simulink model "PSK8_DigitalBandpassComm"  (R2019b)
settings: Solver=VariableStepAuto  StartTime=0.0  StopTime=1e-2  RelTol=1e-3
libraries: commutil2 x2, dspsrcs4 x2, commdigbbndpm3 x2, commfilt2 x2, commchan3 x1, commsink2 x1, commrandsrc3 x1
settings Model: Creator=SEFA  LastModifiedBy=SEFA

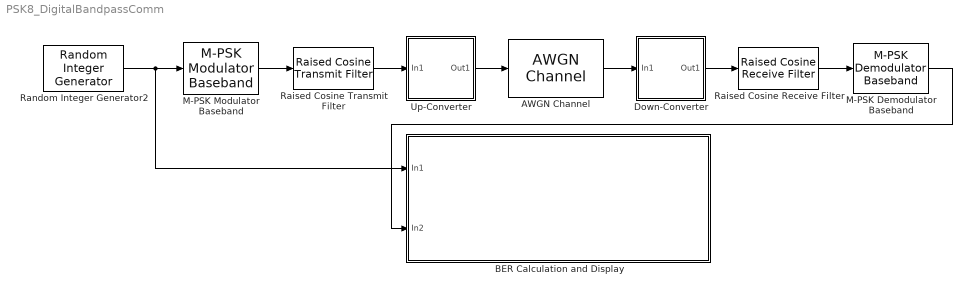
== system PSK8_DigitalBandpassComm ==
  AWGN Channel : commchan3/AWGN Channel  InputProcessing=Columns as channels (frame based)  seed=67  noiseMode="Signal to noise ratio  (Es/No)"  EbNodB=10  EsNodB=SNR  SNRdB=10  bitsPerSym=1  Ps=1/(16)  Tsym=1e-6  variance=1
      settings: SourceProductName=Communications Toolbox
  BER Calculation and Display : Subsystem
  Down-Converter : Subsystem
  M-PSK Demodulator Baseband : commdigbbndpm3/M-PSK Demodulator Baseband  M=8  OutType=Integer  DecType=Hard decision  VarSource=Dialog  Variance=1  Dec=Gray  Mapping=[0:7]  Ph=0  outDtype1=Inherit via internal rule  outDtype2=Inherit via internal rule  derotateFactorWordLen=16  derotateFactorDataTypeStr=Inherit: Same word length as input  derotateFactorLastDataTypeStr=Inherit: Same word length as input
      settings: SourceProductName=Communications Toolbox
  M-PSK Modulator Baseband : commdigbbndpm3/M-PSK Modulator Baseband  M=8  InType=Integer  Enc=Gray  Mapping=[0:7]  Ph=0  outDtype=double  outWordLen=16  outUDDataType=sfix(16)  outFracLenMode=Best precision  outFracLen=15  outDataTypeStr=double  outLastDataTypeStr=double
      settings: SourceProductName=Communications Toolbox
  Raised Cosine Receive Filter : commfilt2/Raised Cosine Receive Filter  filtType=Square root  R=0.2  filtSpan=10  N=8  downFactor=8  downOffset=0  filterGain=2  RateOptions=Allow multirate processing  framing=Mute  checkCoeff=off  variableName=rcRxFilt  currentFiltSpan=10  D=(10)/2  inputOffset=0  sampMode=Mute  saveAsFlag=0  rateMode=Downsampling  checkGain=Normalized  launchFVT=on  roundingMode=Floor  overflowMode=off  coeffDataTypeStr=Inherit: Same word length as input  coeffMin=[]  coeffMax=[]  coeffLastDataTypeStr=Inherit: Same word length as input  accumDataTypeStr=Inherit: Same as product output  accumLastDataTypeStr=Inherit: Same as product output  outputDataTypeStr=Inherit: Same as accumulator  outputMin=[]  outputMax=[]  outputLastDataTypeStr=Inherit: Same as accumulator
      settings: SourceProductName=Communications Toolbox
  Raised Cosine Transmit Filter : commfilt2/Raised Cosine Transmit Filter  filtType=Square root  R=0.2  filtSpan=10  N=8  filterGain=1  RateOptions=Allow multirate processing  framing=Mute  checkCoeff=off  variableName=rcTxFilt  checkGain=Normalized  sampMode=Mute  saveAsFlag=0  currentFiltSpan=10  D=(10)/2  launchFVT=on  roundingMode=Floor  overflowMode=off  coeffDataTypeStr=Inherit: Same word length as input  coeffMin=[]  coeffMax=[]  coeffLastDataTypeStr=Inherit: Same word length as input  outputDataTypeStr=Inherit: Same as accumulator  outputMin=[]  outputMax=[]  outputLastDataTypeStr=Inherit: Same as accumulator
      settings: SourceProductName=Communications Toolbox
  Random Integer Generator2 : commrandsrc3/Random Integer Generator  SetSize=8  SeedSource=Auto  Seed=0  SampleTime=1e-6  SamplesPerFrame=1  OutputDataType=double  SimulateUsing=Interpreted execution
      settings: SourceProductName=Communications Toolbox
  Up-Converter : Subsystem
  wires:
  Down-Converter/1(Out1) -> Raised Cosine Receive Filter/1
  M-PSK Modulator Baseband/1 -> Raised Cosine Transmit Filter/1
  AWGN Channel/1 -> Down-Converter/1(In1)
  Raised Cosine Receive Filter/1 -> M-PSK Demodulator Baseband/1
  M-PSK Demodulator Baseband/1 -> BER Calculation and Display/2(In2)
  Up-Converter/1(Out1) -> AWGN Channel/1
  Random Integer Generator2/1 -> M-PSK Modulator Baseband/1, BER Calculation and Display/1(In1)
  Raised Cosine Transmit Filter/1 -> Up-Converter/1(In1)

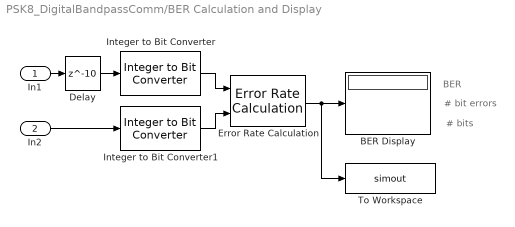
== system PSK8_DigitalBandpassComm/BER Calculation and Display ==
  note: # bit errors
  note: # bits
  note: BER
  In1 : Inport
  In2 : Inport  Port=2
  BER Display : Display
  Delay : Delay  DelayLength=10  InitialCondition=0
  Error Rate Calculation : commsink2/Error Rate Calculation  N=0  st_delay=30  cp_mode=Entire frame  subframe=[]  PMode=Port  WsName=ErrorVec  RsMode2=off  stop=off  numErr=100  maxBits=1e6
      settings: SourceProductName=Communications Toolbox
  Integer to Bit Converter : commutil2/Integer to Bit Converter  nbits=3  signedInputValues=Unsigned  bitOrder=MSB first  outDtype=Inherit via internal rule
      settings: SourceProductName=Communications Toolbox
  Integer to Bit Converter1 : commutil2/Integer to Bit Converter  nbits=3  signedInputValues=Unsigned  bitOrder=MSB first  outDtype=Inherit via internal rule
      settings: SourceProductName=Communications Toolbox
  To Workspace : ToWorkspace  VariableName=simout  SaveFormat=Timeseries  SampleTime=-1
  wires:
  Error Rate Calculation/1 -> To Workspace/1, BER Display/1
  Integer to Bit Converter/1 -> Error Rate Calculation/1
  Integer to Bit Converter1/1 -> Error Rate Calculation/2
  In2/1 -> Integer to Bit Converter1/1
  In1/1 -> Delay/1
  Delay/1 -> Integer to Bit Converter/1

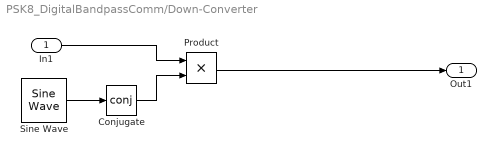
== system PSK8_DigitalBandpassComm/Down-Converter ==
  In1 : Inport
  Conjugate : Math  Operator=conj  RndMeth=Zero  SaturateOnIntegerOverflow=on
  Product : Product
  Sine Wave : dspsrcs4/Sine Wave  Amplitude=1  Frequency=2.5e6  Phase=0  SampleMode=Discrete  OutComplex=Complex  CompMethod=Trigonometric fcn  TableSize=Speed  SampleTime=(1e-6)/8  SamplesPerFrame=1  ResetState=Restart at time zero  OutputFrames=off  dataType=double  wordLen=16  udDataType=sfix(16)  fracBitsMode=Best precision  numFracBits=15  OutDataTypeStr=double  LastOutDataTypeStr=double
  Out1 : Outport
  wires:
  Sine Wave/1 -> Conjugate/1
  In1/1 -> Product/1
  Conjugate/1 -> Product/2
  Product/1 -> Out1/1

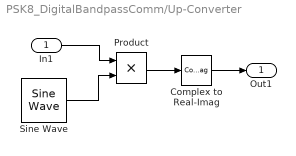
== system PSK8_DigitalBandpassComm/Up-Converter ==
  In1 : Inport
  Complex to Real-Imag : ComplexToRealImag  Output=Real
  Product : Product
  Sine Wave : dspsrcs4/Sine Wave  Amplitude=1  Frequency=2.5e6  Phase=0  SampleMode=Discrete  OutComplex=Complex  CompMethod=Trigonometric fcn  TableSize=Speed  SampleTime=(1e-6)/8  SamplesPerFrame=1  ResetState=Restart at time zero  OutputFrames=off  dataType=double  wordLen=16  udDataType=sfix(16)  fracBitsMode=Best precision  numFracBits=15  OutDataTypeStr=double  LastOutDataTypeStr=double
  Out1 : Outport
  wires:
  Sine Wave/1 -> Product/2
  Product/1 -> Complex to Real-Imag/1
  In1/1 -> Product/1
  Complex to Real-Imag/1 -> Out1/1
